simulink library "LIB_RTCP_DIE_UG_V1_0"  (R2021a)
settings: Solver=VariableStepAuto  StartTime=0.0  StopTime=10.0  RelTol=1e-3
undefined symbols (not defined in the file): DiscIntNeverNeededParam
libraries: c2802xlib x22, c28004xlib x10, pid_lib x2, spsAlphaBetaZerotodq0Lib x1, eeGeneralControl x1, eeStairGenerator x1
settings Model: Creator=luram  LastModifiedBy=luram

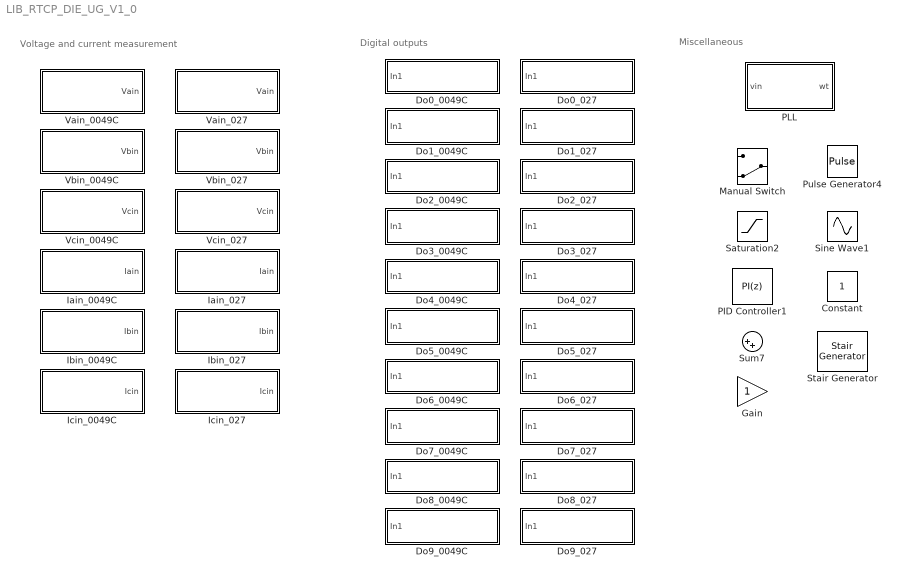
== system LIB_RTCP_DIE_UG_V1_0 ==
  note: Miscellaneous
  note: Digital outputs
  note: Voltage and current measurement
  Constant : Constant
  Do0_0049C : Subsystem
      mask Display: disp('\muC (boolean) --> Dout', 'texmode','on')
  Do0_027 : Subsystem
      mask Display: disp('\muC (boolean) --> Dout', 'texmode','on')
  Do1_0049C : Subsystem
      mask Display: disp('\muC (boolean) --> Dout', 'texmode','on')
  Do1_027 : Subsystem
      mask Display: disp('\muC (boolean) --> Dout', 'texmode','on')
  Do2_0049C : Subsystem
      mask Display: disp('\muC (boolean) --> Dout', 'texmode','on')
  Do2_027 : Subsystem
      mask Display: disp('\muC (boolean) --> Dout', 'texmode','on')
  Do3_0049C : Subsystem
      mask Display: disp('\muC (boolean) --> Dout', 'texmode','on')
  Do3_027 : Subsystem
      mask Display: disp('\muC (boolean) --> Dout', 'texmode','on')
  Do4_0049C : Subsystem
      mask Display: disp('\muC (boolean) --> Dout', 'texmode','on')
  Do4_027 : Subsystem
      mask Display: disp('\muC (boolean) --> Dout', 'texmode','on')
  Do5_0049C : Subsystem
      mask Display: disp('\muC (boolean) --> Dout', 'texmode','on')
  Do5_027 : Subsystem
      mask Display: disp('\muC (boolean) --> Dout', 'texmode','on')
  Do6_0049C : Subsystem
      mask Display: disp('\muC (boolean) --> Dout', 'texmode','on')
  Do6_027 : Subsystem
      mask Display: disp('\muC (boolean) --> Dout', 'texmode','on')
  Do7_0049C : Subsystem
      mask Display: disp('\muC (boolean) --> Dout', 'texmode','on')
  Do7_027 : Subsystem
      mask Display: disp('\muC (boolean) --> Dout', 'texmode','on')
  Do8_0049C : Subsystem
      mask Display: disp('\muC (boolean) --> Dout', 'texmode','on')
  Do8_027 : Subsystem
      mask Display: disp('\muC (boolean) --> Dout', 'texmode','on')
  Do9_0049C : Subsystem
      mask Display: disp('\muC (boolean) --> Dout', 'texmode','on')
  Do9_027 : Subsystem
      mask Display: disp('\muC (boolean) --> Dout', 'texmode','on')
  Gain : Gain
  Iain_0049C : Subsystem  mask(Voltage sensor){Off=0.15, AQPSv=50, Ts=1e-4}
      mask prompts: Off "Offset"; AQPSv "Adquisition"
      mask help:
      | R1=330;
      | R2=300e3;
      | Gain=8.2;
      | R2d=2000;
      | R1d=3000;
      |
      | GananciaAnV=R2d/R1d*Gain*R1/(R1+R2);
      | VtoD=GananciaAnV*4096/3.3;
      | DtoV=1/VtoD;
      mask init:
      | Gain=8.2;
      | R2d=2000;
      | R1d=3000;
      | 
      | Rs=0.02;
      | GananciaAnI=R2d/R1d*Gain*Rs;
      | ItoD=GananciaAnI*4096/3.3;
      | DtoI=1/ItoD;
      mask Help:
      | R1=330;
      | R2=300e3;
      | Gain=8.2;
      | R2d=2000;
      | R1d=3000;
      | 
      | GananciaAnV=R2d/R1d*Gain*R1/(R1+R2);
      | VtoD=GananciaAnV*4096/3.3;
      | DtoV=1/VtoD;
      mask Display: disp('Iin  --> \muC (single) ', 'texmode','on')
  Iain_027 : Subsystem  mask(Voltage sensor){Off=0.15, AQPSv=50, Ts=1e-4}
      mask prompts: Off "Offset"; AQPSv "Adquisition"
      mask help:
      | R1=330;
      | R2=300e3;
      | Gain=8.2;
      | R2d=2000;
      | R1d=3000;
      |
      | GananciaAnV=R2d/R1d*Gain*R1/(R1+R2);
      | VtoD=GananciaAnV*4096/3.3;
      | DtoV=1/VtoD;
      mask init:
      | Gain=8.2;
      | R2d=2000;
      | R1d=3000;
      | 
      | Rs=0.02;
      | GananciaAnI=R2d/R1d*Gain*Rs;
      | ItoD=GananciaAnI*4096/3.3;
      | DtoI=1/ItoD;
      mask Help:
      | R1=330;
      | R2=300e3;
      | Gain=8.2;
      | R2d=2000;
      | R1d=3000;
      | 
      | GananciaAnV=R2d/R1d*Gain*R1/(R1+R2);
      | VtoD=GananciaAnV*4096/3.3;
      | DtoV=1/VtoD;
      mask Display: disp('Iin  --> \muC (single) ', 'texmode','on')
  Ibin_0049C : Subsystem  mask(Voltage sensor){Off=0.15, AQPSv=50, Ts=1e-4}
      mask prompts: Off "Offset"; AQPSv "Adquisition"
      mask help:
      | R1=330;
      | R2=300e3;
      | Gain=8.2;
      | R2d=2000;
      | R1d=3000;
      |
      | GananciaAnV=R2d/R1d*Gain*R1/(R1+R2);
      | VtoD=GananciaAnV*4096/3.3;
      | DtoV=1/VtoD;
      mask init:
      | Gain=8.2;
      | R2d=2000;
      | R1d=3000;
      | 
      | Rs=0.02;
      | GananciaAnI=R2d/R1d*Gain*Rs;
      | ItoD=GananciaAnI*4096/3.3;
      | DtoI=1/ItoD;
      mask Help:
      | R1=330;
      | R2=300e3;
      | Gain=8.2;
      | R2d=2000;
      | R1d=3000;
      | 
      | GananciaAnV=R2d/R1d*Gain*R1/(R1+R2);
      | VtoD=GananciaAnV*4096/3.3;
      | DtoV=1/VtoD;
      mask Display: disp('Iin  --> \muC (single) ', 'texmode','on')
  Ibin_027 : Subsystem  mask(Voltage sensor){Off=0.15, AQPSv=50, Ts=1e-4}
      mask prompts: Off "Offset"; AQPSv "Adquisition"
      mask help:
      | R1=330;
      | R2=300e3;
      | Gain=8.2;
      | R2d=2000;
      | R1d=3000;
      |
      | GananciaAnV=R2d/R1d*Gain*R1/(R1+R2);
      | VtoD=GananciaAnV*4096/3.3;
      | DtoV=1/VtoD;
      mask init:
      | Gain=8.2;
      | R2d=2000;
      | R1d=3000;
      | 
      | Rs=0.02;
      | GananciaAnI=R2d/R1d*Gain*Rs;
      | ItoD=GananciaAnI*4096/3.3;
      | DtoI=1/ItoD;
      mask Help:
      | R1=330;
      | R2=300e3;
      | Gain=8.2;
      | R2d=2000;
      | R1d=3000;
      | 
      | GananciaAnV=R2d/R1d*Gain*R1/(R1+R2);
      | VtoD=GananciaAnV*4096/3.3;
      | DtoV=1/VtoD;
      mask Display: disp('Iin  --> \muC (single) ', 'texmode','on')
  Icin_0049C : Subsystem  mask(Voltage sensor){Off=0.15, AQPSv=50, Ts=1e-4}
      mask prompts: Off "Offset"; AQPSv "Adquisition"
      mask help:
      | R1=330;
      | R2=300e3;
      | Gain=8.2;
      | R2d=2000;
      | R1d=3000;
      |
      | GananciaAnV=R2d/R1d*Gain*R1/(R1+R2);
      | VtoD=GananciaAnV*4096/3.3;
      | DtoV=1/VtoD;
      mask init:
      | Gain=8.2;
      | R2d=2000;
      | R1d=3000;
      | 
      | Rs=0.02;
      | GananciaAnI=R2d/R1d*Gain*Rs;
      | ItoD=GananciaAnI*4096/3.3;
      | DtoI=1/ItoD;
      mask Help:
      | R1=330;
      | R2=300e3;
      | Gain=8.2;
      | R2d=2000;
      | R1d=3000;
      | 
      | GananciaAnV=R2d/R1d*Gain*R1/(R1+R2);
      | VtoD=GananciaAnV*4096/3.3;
      | DtoV=1/VtoD;
      mask Display: disp('Iin  --> \muC (single) ', 'texmode','on')
  Icin_027 : Subsystem  mask(Voltage sensor){Off=0.15, AQPSv=50, Ts=1e-4}
      mask prompts: Off "Offset"; AQPSv "Adquisition"
      mask help:
      | R1=330;
      | R2=300e3;
      | Gain=8.2;
      | R2d=2000;
      | R1d=3000;
      |
      | GananciaAnV=R2d/R1d*Gain*R1/(R1+R2);
      | VtoD=GananciaAnV*4096/3.3;
      | DtoV=1/VtoD;
      mask init:
      | Gain=8.2;
      | R2d=2000;
      | R1d=3000;
      | 
      | Rs=0.02;
      | GananciaAnI=R2d/R1d*Gain*Rs;
      | ItoD=GananciaAnI*4096/3.3;
      | DtoI=1/ItoD;
      mask Help:
      | R1=330;
      | R2=300e3;
      | Gain=8.2;
      | R2d=2000;
      | R1d=3000;
      | 
      | GananciaAnV=R2d/R1d*Gain*R1/(R1+R2);
      | VtoD=GananciaAnV*4096/3.3;
      | DtoV=1/VtoD;
      mask Display: disp('Iin  --> \muC (single) ', 'texmode','on')
  Manual Switch : ManualSwitch  CurrentSetting=0
  PID Controller1 : pid_lib/PID Controller  Controller=PI  Form=Parallel  TimeDomain=Discrete-time  UseExternalTs=off  SampleTime=1e-5  IntegratorMethod=Forward Euler  FilterMethod=Forward Euler  ControllerParametersSource=internal  P=1  I=1  D=0  UseFilter=on  N=100  TunerSelectOption=Transfer Function Based (PID Tuner App)  InitialConditionSource=internal  InitialConditionForIntegrator=0  InitialConditionForFilter=0  DifferentiatorICPrevScaledInput=0  ExternalReset=none  TrackingMode=off  Kt=1  LimitOutput=on  SatLimitsSource=internal  UpperSaturationLimit=1  LowerSaturationLimit=-1  LinearizeAsGain=on  AntiWindupMode=none  Kb=1  POutMin=[]  POutMax=[]  IOutMin=[]  IOutMax=[]  DOutMin=[]  DOutMax=[]  NOutMin=[]  NOutMax=[]  SumOutMin=[]  SumOutMax=[]  SaturationOutMin=[]  SaturationOutMax=[]  PParamMin=[]  PParamMax=[]  IParamMin=[]  IParamMax=[]  DParamMin=[]  DParamMax=[]  NParamMin=[]  NParamMax=[]  KbParamMin=[]  KbParamMax=[]  KtParamMin=[]  KtParamMax=[]  KbOutMin=[]  KbOutMax=[]  KtOutMin=[]  KtOutMax=[]  IntegratorOutMin=[]  IntegratorOutMax=[]  FilterOutMin=[]  FilterOutMax=[]  SumI1OutMin=[]  SumI1OutMax=[]  SumI2OutMin=[]  SumI2OutMax=[]  SumI3OutMin=[]  SumI3OutMax=[]  SumI4OutMin=[]  SumI4OutMax=[]  SumDOutMin=[]  SumDOutMax=[]  DifferentiatorOutMin=[]  DifferentiatorOutMax=[]  FilterDiffOutCoefMin=[]  FilterDiffOutCoefMax=[]  ReciprocalOutMin=[]  ReciprocalOutMax=[]  SumDenOutMin=[]  SumDenOutMax=[]  SumNumOutMin=[]  SumNumOutMax=[]  DivideOutMin=[]  DivideOutMax=[]  UdiffTsProdOutMin=[]  UdiffTsProdOutMax=[]  NTsProdOutMin=[]  NTsProdOutMax=[]  UintegralTsProdOutMin=[]  UintegralTsProdOutMax=[]  UngainTsProdOutMin=[]  UngainTsProdOutMax=[]  IntegratorContinuousStateAttributes=''  IntegratorStateMustResolveToSignalObject=off  IntegratorRTWStateStorageClass=Auto  FilterContinuousStateAttributes=''  FilterStateMustResolveToSignalObject=off  FilterRTWStateStorageClass=Auto  ParallelPVariant=InternalParameters  IdealPVariant=Disabled  IVariant=InternalParameters  DVariant=Disabled  IntegratorVariant=Discrete  SatVariant=Enabled  AWVariant=Passthrough  PCopyVariant=Disabled  TRVariant=Disabled  FdbkBlocksVariant=Forward  IdealPFdbkVariant=Disabled  SatFdbkVariant=Disabled  DerivativeFilterVariant=Disabled  NVariant=Disabled  NCopyVariant=Disabled_SignalSpec  FilterICVariant=Disabled  IntegratorICVariant=InternalICs  ExternalResetVariant=Disabled  TRSumVariant=Passthrough  SumFdbkVariant=Disabled  SumVariant=Sum_PI  TsampFilterVariant=InternalTs  TsampNgainVariant=Passthrough  TsampIntegralVariant=Passthrough  ExternalSaturationOutDataTypeStr=Inherit: Same as second input
  PLL : Subsystem  mask{Ffun=60, Ts=-1}
      mask prompts: Ffun "Fundamental Frequency"
      mask Display: disp('In  --> wt ', 'texmode','on')
  Pulse Generator4 : DiscretePulseGenerator  PulseType=Time based  Period=0.6  PulseWidth=50
  Saturation2 : Saturate  UpperLimit=4900  LowerLimit=100
  Sine Wave1 : Sin  Frequency=2*pi*60
  Stair Generator : eeStairGenerator/Stair Generator  LabelModeActiveChoice=Discrete  TimeInput=[0.5 1 3 3.5]  AmplitudeInput=[1 -1 2.5 0]  SampleTime=-1  RepeatPattern=off  OutDataTypeStr=double
      settings: SourceProductBaseCode=PS
  Sum7 : Sum  Inputs=|++
  Vain_0049C : Subsystem  mask(Voltage sensor){Off=3, AQPSv=50, Ts=1e-4}
      mask prompts: Off "Offset"; AQPSv "Adquisition"
      mask help:
      | R1=330;
      | R2=300e3;
      | Gain=8.2;
      | R2d=2000;
      | R1d=3000;
      |
      | GananciaAnV=R2d/R1d*Gain*R1/(R1+R2);
      | VtoD=GananciaAnV*4096/3.3;
      | DtoV=1/VtoD;
      mask init:
      | R1=330;
      | R2=300e3;
      | Gain=8.2;
      | R2d=2000;
      | R1d=3000;
      | 
      | GananciaAnV=R2d/R1d*Gain*R1/(R1+R2);
      | VtoD=GananciaAnV*4096/3.3;
      | DtoV=1/VtoD;
      mask Help:
      | R1=330;
      | R2=300e3;
      | Gain=8.2;
      | R2d=2000;
      | R1d=3000;
      | 
      | GananciaAnV=R2d/R1d*Gain*R1/(R1+R2);
      | VtoD=GananciaAnV*4096/3.3;
      | DtoV=1/VtoD;
      mask Display: disp('Vin  --> \muC (single) ', 'texmode','on')
  Vain_027 : Subsystem  mask(Voltage sensor){Off=3, AQPSv=50, Ts=1e-4}
      mask prompts: Off "Offset"; AQPSv "Adquisition"
      mask help:
      | R1=330;
      | R2=300e3;
      | Gain=8.2;
      | R2d=2000;
      | R1d=3000;
      |
      | GananciaAnV=R2d/R1d*Gain*R1/(R1+R2);
      | VtoD=GananciaAnV*4096/3.3;
      | DtoV=1/VtoD;
      mask init:
      | R1=330;
      | R2=300e3;
      | Gain=8.2;
      | R2d=2000;
      | R1d=3000;
      | 
      | GananciaAnV=R2d/R1d*Gain*R1/(R1+R2);
      | VtoD=GananciaAnV*4096/3.3;
      | DtoV=1/VtoD;
      mask Help:
      | R1=330;
      | R2=300e3;
      | Gain=8.2;
      | R2d=2000;
      | R1d=3000;
      | 
      | GananciaAnV=R2d/R1d*Gain*R1/(R1+R2);
      | VtoD=GananciaAnV*4096/3.3;
      | DtoV=1/VtoD;
      mask Display: disp('Vin  --> \muC (single) ', 'texmode','on')
  Vbin_0049C : Subsystem  mask{Off=3, AQPSv=50, Ts=1e-4}
      mask prompts: Off "Offset"; AQPSv "Adquisition"
      mask init:
      | R1=330;
      | R2=300e3;
      | Gain=8.2;
      | R2d=2000;
      | R1d=3000;
      | 
      | GananciaAnV=R2d/R1d*Gain*R1/(R1+R2);
      | VtoD=GananciaAnV*4096/3.3;
      | DtoV=1/VtoD;
      mask Display: disp('Vin  --> \muC (single) ', 'texmode','on')
  Vbin_027 : Subsystem  mask{Off=3, AQPSv=50, Ts=1e-4}
      mask prompts: Off "Offset"; AQPSv "Adquisition"
      mask init:
      | R1=330;
      | R2=300e3;
      | Gain=8.2;
      | R2d=2000;
      | R1d=3000;
      | 
      | GananciaAnV=R2d/R1d*Gain*R1/(R1+R2);
      | VtoD=GananciaAnV*4096/3.3;
      | DtoV=1/VtoD;
      mask Display: disp('Vin  --> \muC (single) ', 'texmode','on')
  Vcin_0049C : Subsystem  mask{Off=3, AQPSv=50, Ts=1e-4}
      mask prompts: Off "Offset"; AQPSv "Adquisition"
      mask init:
      | R1=330;
      | R2=300e3;
      | Gain=8.2;
      | R2d=2000;
      | R1d=3000;
      | 
      | GananciaAnV=R2d/R1d*Gain*R1/(R1+R2);
      | VtoD=GananciaAnV*4096/3.3;
      | DtoV=1/VtoD;
      mask Display: disp('Vin  --> \muC (single) ', 'texmode','on')
  Vcin_027 : Subsystem  mask{Off=3, AQPSv=50, Ts=1e-4}
      mask prompts: Off "Offset"; AQPSv "Adquisition"
      mask init:
      | R1=330;
      | R2=300e3;
      | Gain=8.2;
      | R2d=2000;
      | R1d=3000;
      | 
      | GananciaAnV=R2d/R1d*Gain*R1/(R1+R2);
      | VtoD=GananciaAnV*4096/3.3;
      | DtoV=1/VtoD;
      mask Display: disp('Vin  --> \muC (single) ', 'texmode','on')

== system LIB_RTCP_DIE_UG_V1_0/Do0_0049C ==
  In1 : Inport
  Digital Output : c28004xlib/Digital Output  GPIO_Number=GPIO8~GPIO15  GPIO_Bit0=off  GPIO_BIT0_Toggle=off  GPIO_Bit1=off  GPIO_BIT1_Toggle=off  GPIO_Bit2=on  GPIO_BIT2_Toggle=off  GPIO_Bit3=off  GPIO_BIT3_Toggle=off  GPIO_Bit4=off  GPIO_BIT4_Toggle=off  GPIO_Bit5=off  GPIO_BIT5_Toggle=off  GPIO_Bit6=off  GPIO_BIT6_Toggle=off  GPIO_Bit7=off  GPIO_BIT7_Toggle=off
      settings: SourceProductBaseCode=TIC2000
  wires:
  In1/1 -> Digital Output/1

== system LIB_RTCP_DIE_UG_V1_0/Do0_027 ==
  In1 : Inport
  Digital Output : c2802xlib/Digital Output  GPIO_Number=GPIO0~GPIO7  GPIO_Bit0=on  GPIO_BIT0_Toggle=off  GPIO_Bit1=off  GPIO_BIT1_Toggle=off  GPIO_Bit2=off  GPIO_BIT2_Toggle=off  GPIO_Bit3=off  GPIO_BIT3_Toggle=off  GPIO_Bit4=off  GPIO_BIT4_Toggle=off  GPIO_Bit5=off  GPIO_BIT5_Toggle=off  GPIO_Bit6=off  GPIO_BIT6_Toggle=off  GPIO_Bit7=off  GPIO_BIT7_Toggle=off
      settings: SourceProductBaseCode=TIC2000
  wires:
  In1/1 -> Digital Output/1

== system LIB_RTCP_DIE_UG_V1_0/Do1_0049C ==
  In1 : Inport
  Digital Output : c28004xlib/Digital Output  GPIO_Number=GPIO8~GPIO15  GPIO_Bit0=off  GPIO_BIT0_Toggle=off  GPIO_Bit1=off  GPIO_BIT1_Toggle=off  GPIO_Bit2=off  GPIO_BIT2_Toggle=off  GPIO_Bit3=on  GPIO_BIT3_Toggle=off  GPIO_Bit4=off  GPIO_BIT4_Toggle=off  GPIO_Bit5=off  GPIO_BIT5_Toggle=off  GPIO_Bit6=off  GPIO_BIT6_Toggle=off  GPIO_Bit7=off  GPIO_BIT7_Toggle=off
      settings: SourceProductBaseCode=TIC2000
  wires:
  In1/1 -> Digital Output/1

== system LIB_RTCP_DIE_UG_V1_0/Do1_027 ==
  In1 : Inport
  Digital Output : c2802xlib/Digital Output  GPIO_Number=GPIO0~GPIO7  GPIO_Bit0=off  GPIO_BIT0_Toggle=off  GPIO_Bit1=on  GPIO_BIT1_Toggle=off  GPIO_Bit2=off  GPIO_BIT2_Toggle=off  GPIO_Bit3=off  GPIO_BIT3_Toggle=off  GPIO_Bit4=off  GPIO_BIT4_Toggle=off  GPIO_Bit5=off  GPIO_BIT5_Toggle=off  GPIO_Bit6=off  GPIO_BIT6_Toggle=off  GPIO_Bit7=off  GPIO_BIT7_Toggle=off
      settings: SourceProductBaseCode=TIC2000
  wires:
  In1/1 -> Digital Output/1

== system LIB_RTCP_DIE_UG_V1_0/Do2_0049C ==
  In1 : Inport
  Digital Output : c28004xlib/Digital Output  GPIO_Number=GPIO8~GPIO15  GPIO_Bit0=on  GPIO_BIT0_Toggle=off  GPIO_Bit1=off  GPIO_BIT1_Toggle=off  GPIO_Bit2=off  GPIO_BIT2_Toggle=off  GPIO_Bit3=off  GPIO_BIT3_Toggle=off  GPIO_Bit4=off  GPIO_BIT4_Toggle=off  GPIO_Bit5=off  GPIO_BIT5_Toggle=off  GPIO_Bit6=off  GPIO_BIT6_Toggle=off  GPIO_Bit7=off  GPIO_BIT7_Toggle=off
      settings: SourceProductBaseCode=TIC2000
  wires:
  In1/1 -> Digital Output/1

== system LIB_RTCP_DIE_UG_V1_0/Do2_027 ==
  In1 : Inport
  Digital Output : c2802xlib/Digital Output  GPIO_Number=GPIO0~GPIO7  GPIO_Bit0=off  GPIO_BIT0_Toggle=off  GPIO_Bit1=off  GPIO_BIT1_Toggle=off  GPIO_Bit2=on  GPIO_BIT2_Toggle=off  GPIO_Bit3=off  GPIO_BIT3_Toggle=off  GPIO_Bit4=off  GPIO_BIT4_Toggle=off  GPIO_Bit5=off  GPIO_BIT5_Toggle=off  GPIO_Bit6=off  GPIO_BIT6_Toggle=off  GPIO_Bit7=off  GPIO_BIT7_Toggle=off
      settings: SourceProductBaseCode=TIC2000
  wires:
  In1/1 -> Digital Output/1

== system LIB_RTCP_DIE_UG_V1_0/Do3_0049C ==
  In1 : Inport
  Digital Output : c28004xlib/Digital Output  GPIO_Number=GPIO8~GPIO15  GPIO_Bit0=off  GPIO_BIT0_Toggle=off  GPIO_Bit1=on  GPIO_BIT1_Toggle=off  GPIO_Bit2=off  GPIO_BIT2_Toggle=off  GPIO_Bit3=off  GPIO_BIT3_Toggle=off  GPIO_Bit4=off  GPIO_BIT4_Toggle=off  GPIO_Bit5=off  GPIO_BIT5_Toggle=off  GPIO_Bit6=off  GPIO_BIT6_Toggle=off  GPIO_Bit7=off  GPIO_BIT7_Toggle=off
      settings: SourceProductBaseCode=TIC2000
  wires:
  In1/1 -> Digital Output/1

== system LIB_RTCP_DIE_UG_V1_0/Do3_027 ==
  In1 : Inport
  Digital Output : c2802xlib/Digital Output  GPIO_Number=GPIO0~GPIO7  GPIO_Bit0=off  GPIO_BIT0_Toggle=off  GPIO_Bit1=off  GPIO_BIT1_Toggle=off  GPIO_Bit2=off  GPIO_BIT2_Toggle=off  GPIO_Bit3=on  GPIO_BIT3_Toggle=off  GPIO_Bit4=off  GPIO_BIT4_Toggle=off  GPIO_Bit5=off  GPIO_BIT5_Toggle=off  GPIO_Bit6=off  GPIO_BIT6_Toggle=off  GPIO_Bit7=off  GPIO_BIT7_Toggle=off
      settings: SourceProductBaseCode=TIC2000
  wires:
  In1/1 -> Digital Output/1

== system LIB_RTCP_DIE_UG_V1_0/Do4_0049C ==
  In1 : Inport
  Digital Output : c28004xlib/Digital Output  GPIO_Number=GPIO0~GPIO7  GPIO_Bit0=off  GPIO_BIT0_Toggle=off  GPIO_Bit1=off  GPIO_BIT1_Toggle=off  GPIO_Bit2=off  GPIO_BIT2_Toggle=off  GPIO_Bit3=off  GPIO_BIT3_Toggle=off  GPIO_Bit4=on  GPIO_BIT4_Toggle=off  GPIO_Bit5=off  GPIO_BIT5_Toggle=off  GPIO_Bit6=off  GPIO_BIT6_Toggle=off  GPIO_Bit7=off  GPIO_BIT7_Toggle=off
      settings: SourceProductBaseCode=TIC2000
  wires:
  In1/1 -> Digital Output/1

== system LIB_RTCP_DIE_UG_V1_0/Do4_027 ==
  In1 : Inport
  Digital Output : c2802xlib/Digital Output  GPIO_Number=GPIO0~GPIO7  GPIO_Bit0=off  GPIO_BIT0_Toggle=off  GPIO_Bit1=off  GPIO_BIT1_Toggle=off  GPIO_Bit2=off  GPIO_BIT2_Toggle=off  GPIO_Bit3=off  GPIO_BIT3_Toggle=off  GPIO_Bit4=on  GPIO_BIT4_Toggle=off  GPIO_Bit5=off  GPIO_BIT5_Toggle=off  GPIO_Bit6=off  GPIO_BIT6_Toggle=off  GPIO_Bit7=off  GPIO_BIT7_Toggle=off
      settings: SourceProductBaseCode=TIC2000
  wires:
  In1/1 -> Digital Output/1

== system LIB_RTCP_DIE_UG_V1_0/Do5_0049C ==
  In1 : Inport
  Digital Output : c28004xlib/Digital Output  GPIO_Number=GPIO0~GPIO7  GPIO_Bit0=off  GPIO_BIT0_Toggle=off  GPIO_Bit1=off  GPIO_BIT1_Toggle=off  GPIO_Bit2=off  GPIO_BIT2_Toggle=off  GPIO_Bit3=off  GPIO_BIT3_Toggle=off  GPIO_Bit4=off  GPIO_BIT4_Toggle=off  GPIO_Bit5=on  GPIO_BIT5_Toggle=off  GPIO_Bit6=off  GPIO_BIT6_Toggle=off  GPIO_Bit7=off  GPIO_BIT7_Toggle=off
      settings: SourceProductBaseCode=TIC2000
  wires:
  In1/1 -> Digital Output/1

== system LIB_RTCP_DIE_UG_V1_0/Do5_027 ==
  In1 : Inport
  Digital Output : c2802xlib/Digital Output  GPIO_Number=GPIO0~GPIO7  GPIO_Bit0=off  GPIO_BIT0_Toggle=off  GPIO_Bit1=off  GPIO_BIT1_Toggle=off  GPIO_Bit2=off  GPIO_BIT2_Toggle=off  GPIO_Bit3=off  GPIO_BIT3_Toggle=off  GPIO_Bit4=off  GPIO_BIT4_Toggle=off  GPIO_Bit5=on  GPIO_BIT5_Toggle=off  GPIO_Bit6=off  GPIO_BIT6_Toggle=off  GPIO_Bit7=off  GPIO_BIT7_Toggle=off
      settings: SourceProductBaseCode=TIC2000
  wires:
  In1/1 -> Digital Output/1

== system LIB_RTCP_DIE_UG_V1_0/Do6_0049C ==
  In1 : Inport
  Digital Output : c28004xlib/Digital Output  GPIO_Number=GPIO16~GPIO23  GPIO_Bit0=on  GPIO_BIT0_Toggle=off  GPIO_Bit1=off  GPIO_BIT1_Toggle=off  GPIO_Bit2=off  GPIO_BIT2_Toggle=off  GPIO_Bit3=off  GPIO_BIT3_Toggle=off  GPIO_Bit4=off  GPIO_BIT4_Toggle=off  GPIO_Bit5=off  GPIO_BIT5_Toggle=off  GPIO_Bit6=off  GPIO_BIT6_Toggle=off  GPIO_Bit7=off  GPIO_BIT7_Toggle=off
      settings: SourceProductBaseCode=TIC2000
  wires:
  In1/1 -> Digital Output/1

== system LIB_RTCP_DIE_UG_V1_0/Do6_027 ==
  In1 : Inport
  Digital Output : c2802xlib/Digital Output  GPIO_Number=GPIO0~GPIO7  GPIO_Bit0=off  GPIO_BIT0_Toggle=off  GPIO_Bit1=off  GPIO_BIT1_Toggle=off  GPIO_Bit2=off  GPIO_BIT2_Toggle=off  GPIO_Bit3=off  GPIO_BIT3_Toggle=off  GPIO_Bit4=off  GPIO_BIT4_Toggle=off  GPIO_Bit5=off  GPIO_BIT5_Toggle=off  GPIO_Bit6=on  GPIO_BIT6_Toggle=off  GPIO_Bit7=off  GPIO_BIT7_Toggle=off
      settings: SourceProductBaseCode=TIC2000
  wires:
  In1/1 -> Digital Output/1

== system LIB_RTCP_DIE_UG_V1_0/Do7_0049C ==
  In1 : Inport
  Digital Output : c28004xlib/Digital Output  GPIO_Number=GPIO16~GPIO23  GPIO_Bit0=off  GPIO_BIT0_Toggle=off  GPIO_Bit1=on  GPIO_BIT1_Toggle=off  GPIO_Bit2=off  GPIO_BIT2_Toggle=off  GPIO_Bit3=off  GPIO_BIT3_Toggle=off  GPIO_Bit4=off  GPIO_BIT4_Toggle=off  GPIO_Bit5=off  GPIO_BIT5_Toggle=off  GPIO_Bit6=off  GPIO_BIT6_Toggle=off  GPIO_Bit7=off  GPIO_BIT7_Toggle=off
      settings: SourceProductBaseCode=TIC2000
  wires:
  In1/1 -> Digital Output/1

== system LIB_RTCP_DIE_UG_V1_0/Do7_027 ==
  In1 : Inport
  Digital Output : c2802xlib/Digital Output  GPIO_Number=GPIO0~GPIO7  GPIO_Bit0=off  GPIO_BIT0_Toggle=off  GPIO_Bit1=off  GPIO_BIT1_Toggle=off  GPIO_Bit2=off  GPIO_BIT2_Toggle=off  GPIO_Bit3=off  GPIO_BIT3_Toggle=off  GPIO_Bit4=off  GPIO_BIT4_Toggle=off  GPIO_Bit5=off  GPIO_BIT5_Toggle=off  GPIO_Bit6=off  GPIO_BIT6_Toggle=off  GPIO_Bit7=on  GPIO_BIT7_Toggle=off
      settings: SourceProductBaseCode=TIC2000
  wires:
  In1/1 -> Digital Output/1

== system LIB_RTCP_DIE_UG_V1_0/Do8_0049C ==
  In1 : Inport
  Digital Output : c28004xlib/Digital Output  GPIO_Number=GPIO56~GPIO63  GPIO_Bit0=off  GPIO_BIT0_Toggle=off  GPIO_Bit1=off  GPIO_BIT1_Toggle=off  GPIO_Bit2=on  GPIO_BIT2_Toggle=off  GPIO_Bit3=off  GPIO_BIT3_Toggle=off  GPIO_Bit4=off  GPIO_BIT4_Toggle=off  GPIO_Bit5=off  GPIO_BIT5_Toggle=off  GPIO_Bit6=off  GPIO_BIT6_Toggle=off  GPIO_Bit7=off  GPIO_BIT7_Toggle=off
      settings: SourceProductBaseCode=TIC2000
  wires:
  In1/1 -> Digital Output/1

== system LIB_RTCP_DIE_UG_V1_0/Do8_027 ==
  In1 : Inport
  Digital Output : c2802xlib/Digital Output  GPIO_Number=GPIO16~GPIO23  GPIO_Bit0=on  GPIO_BIT0_Toggle=off  GPIO_Bit1=off  GPIO_BIT1_Toggle=off  GPIO_Bit2=off  GPIO_BIT2_Toggle=off  GPIO_Bit3=off  GPIO_BIT3_Toggle=off  GPIO_Bit4=off  GPIO_BIT4_Toggle=off  GPIO_Bit5=off  GPIO_BIT5_Toggle=off  GPIO_Bit6=off  GPIO_BIT6_Toggle=off  GPIO_Bit7=off  GPIO_BIT7_Toggle=off
      settings: SourceProductBaseCode=TIC2000
  wires:
  In1/1 -> Digital Output/1

== system LIB_RTCP_DIE_UG_V1_0/Do9_0049C ==
  In1 : Inport
  Digital Output : c28004xlib/Digital Output  GPIO_Number=GPIO24~GPIO31  GPIO_Bit0=off  GPIO_BIT0_Toggle=off  GPIO_Bit1=off  GPIO_BIT1_Toggle=off  GPIO_Bit2=off  GPIO_BIT2_Toggle=off  GPIO_Bit3=off  GPIO_BIT3_Toggle=off  GPIO_Bit4=off  GPIO_BIT4_Toggle=off  GPIO_Bit5=off  GPIO_BIT5_Toggle=off  GPIO_Bit6=on  GPIO_BIT6_Toggle=off  GPIO_Bit7=off  GPIO_BIT7_Toggle=off
      settings: SourceProductBaseCode=TIC2000
  wires:
  In1/1 -> Digital Output/1

== system LIB_RTCP_DIE_UG_V1_0/Do9_027 ==
  In1 : Inport
  Digital Output : c2802xlib/Digital Output  GPIO_Number=GPIO16~GPIO23  GPIO_Bit0=off  GPIO_BIT0_Toggle=off  GPIO_Bit1=on  GPIO_BIT1_Toggle=off  GPIO_Bit2=off  GPIO_BIT2_Toggle=off  GPIO_Bit3=off  GPIO_BIT3_Toggle=off  GPIO_Bit4=off  GPIO_BIT4_Toggle=off  GPIO_Bit5=off  GPIO_BIT5_Toggle=off  GPIO_Bit6=off  GPIO_BIT6_Toggle=off  GPIO_Bit7=off  GPIO_BIT7_Toggle=off
      settings: SourceProductBaseCode=TIC2000
  wires:
  In1/1 -> Digital Output/1

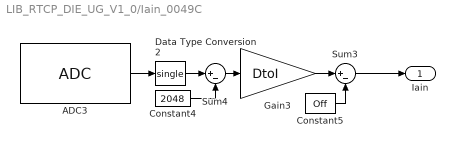
== system LIB_RTCP_DIE_UG_V1_0/Iain_0049C ==
  ADC3 : c2802xlib/ADC  blkParamProc=C2000_Type5  ADCModule=B  samplingMode=Single sample mode  ADCResolution=12-bit (Single-ended input)  useSOC1=SOC1  useSOC2=SOC0_SOC1  SOCAcquisitionWindow=AQPSv  SOCTriggerSource=Software  SOCInterruptTrigger=No ADCINT  Ts=Ts  dType=uint16  postInterrupt=off  interruptSel=ADCINT1  ADCINTContinuous=on  endma=off  chdma=1  conv1=ADCINA0  conv2=ADCINA0 and ADCINB0  conv1_Type4=ADCIN2  conv2_Type4=ADCIN0 and ADCIN1
  Constant4 : Constant  Value=2048
  Constant5 : Constant  Value=Off
  Data Type Conversion2 : DataTypeConversion  OutDataTypeStr=single
  Gain3 : Gain  Gain=DtoI
  Sum3 : Sum  Inputs=|+-
  Sum4 : Sum  Inputs=|+-
  Iain : Outport
  wires:
  Sum4/1 -> Gain3/1
  Sum3/1 -> Iain/1
  Gain3/1 -> Sum3/1
  Constant4/1 -> Sum4/2
  Constant5/1 -> Sum3/2
  Data Type Conversion2/1 -> Sum4/1
  ADC3/1 -> Data Type Conversion2/1

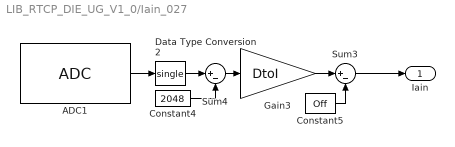
== system LIB_RTCP_DIE_UG_V1_0/Iain_027 ==
  ADC1 : c2802xlib/ADC  blkParamProc=C2000  ADCModule=1  samplingMode=Single sample mode  ADCResolution=12-bit (Single-ended input)  useSOC1=SOC0  useSOC2=SOC0_SOC1  SOCAcquisitionWindow=AQPSv  SOCTriggerSource=Software  SOCInterruptTrigger=No ADCINT  Ts=Ts  dType=uint16  postInterrupt=off  interruptSel=ADCINT1  ADCINTContinuous=on  endma=off  chdma=1  conv1=ADCINB1  conv2=ADCINA0 and ADCINB0  conv1_Type4=ADCIN0  conv2_Type4=ADCIN0 and ADCIN1
  Constant4 : Constant  Value=2048
  Constant5 : Constant  Value=Off
  Data Type Conversion2 : DataTypeConversion  OutDataTypeStr=single
  Gain3 : Gain  Gain=DtoI
  Sum3 : Sum  Inputs=|+-
  Sum4 : Sum  Inputs=|+-
  Iain : Outport
  wires:
  Sum4/1 -> Gain3/1
  Sum3/1 -> Iain/1
  Gain3/1 -> Sum3/1
  Constant4/1 -> Sum4/2
  Constant5/1 -> Sum3/2
  Data Type Conversion2/1 -> Sum4/1
  ADC1/1 -> Data Type Conversion2/1

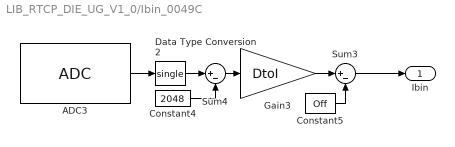
== system LIB_RTCP_DIE_UG_V1_0/Ibin_0049C ==
  ADC3 : c2802xlib/ADC  blkParamProc=C2000_Type5  ADCModule=C  samplingMode=Single sample mode  ADCResolution=12-bit (Single-ended input)  useSOC1=SOC1  useSOC2=SOC0_SOC1  SOCAcquisitionWindow=AQPSv  SOCTriggerSource=Software  SOCInterruptTrigger=No ADCINT  Ts=Ts  dType=uint16  postInterrupt=off  interruptSel=ADCINT1  ADCINTContinuous=on  endma=off  chdma=1  conv1=ADCINA0  conv2=ADCINA0 and ADCINB0  conv1_Type4=ADCIN0  conv2_Type4=ADCIN0 and ADCIN1
  Constant4 : Constant  Value=2048
  Constant5 : Constant  Value=Off
  Data Type Conversion2 : DataTypeConversion  OutDataTypeStr=single
  Gain3 : Gain  Gain=DtoI
  Sum3 : Sum  Inputs=|+-
  Sum4 : Sum  Inputs=|+-
  Ibin : Outport
  wires:
  Sum4/1 -> Gain3/1
  Sum3/1 -> Ibin/1
  Gain3/1 -> Sum3/1
  Constant4/1 -> Sum4/2
  Constant5/1 -> Sum3/2
  Data Type Conversion2/1 -> Sum4/1
  ADC3/1 -> Data Type Conversion2/1

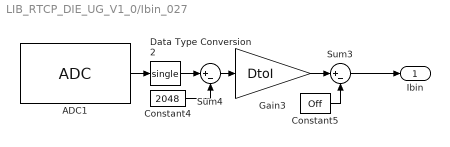
== system LIB_RTCP_DIE_UG_V1_0/Ibin_027 ==
  ADC1 : c2802xlib/ADC  blkParamProc=C2000  ADCModule=1  samplingMode=Single sample mode  ADCResolution=12-bit (Single-ended input)  useSOC1=SOC0  useSOC2=SOC0_SOC1  SOCAcquisitionWindow=AQPSv  SOCTriggerSource=Software  SOCInterruptTrigger=No ADCINT  Ts=Ts  dType=uint16  postInterrupt=off  interruptSel=ADCINT1  ADCINTContinuous=on  endma=off  chdma=1  conv1=ADCINB3  conv2=ADCINA0 and ADCINB0  conv1_Type4=ADCIN0  conv2_Type4=ADCIN0 and ADCIN1
  Constant4 : Constant  Value=2048
  Constant5 : Constant  Value=Off
  Data Type Conversion2 : DataTypeConversion  OutDataTypeStr=single
  Gain3 : Gain  Gain=DtoI
  Sum3 : Sum  Inputs=|+-
  Sum4 : Sum  Inputs=|+-
  Ibin : Outport
  wires:
  Sum4/1 -> Gain3/1
  Sum3/1 -> Ibin/1
  Gain3/1 -> Sum3/1
  Constant4/1 -> Sum4/2
  Constant5/1 -> Sum3/2
  Data Type Conversion2/1 -> Sum4/1
  ADC1/1 -> Data Type Conversion2/1

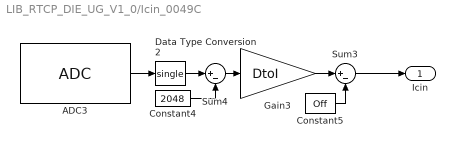
== system LIB_RTCP_DIE_UG_V1_0/Icin_0049C ==
  ADC3 : c2802xlib/ADC  blkParamProc=C2000_Type5  ADCModule=A  samplingMode=Single sample mode  ADCResolution=12-bit (Single-ended input)  useSOC1=SOC1  useSOC2=SOC0_SOC1  SOCAcquisitionWindow=AQPSv  SOCTriggerSource=Software  SOCInterruptTrigger=No ADCINT  Ts=Ts  dType=uint16  postInterrupt=off  interruptSel=ADCINT1  ADCINTContinuous=on  endma=off  chdma=1  conv1=ADCINA0  conv2=ADCINA0 and ADCINB0  conv1_Type4=ADCIN9  conv2_Type4=ADCIN0 and ADCIN1
  Constant4 : Constant  Value=2048
  Constant5 : Constant  Value=Off
  Data Type Conversion2 : DataTypeConversion  OutDataTypeStr=single
  Gain3 : Gain  Gain=DtoI
  Sum3 : Sum  Inputs=|+-
  Sum4 : Sum  Inputs=|+-
  Icin : Outport
  wires:
  Sum4/1 -> Gain3/1
  Sum3/1 -> Icin/1
  Gain3/1 -> Sum3/1
  Constant4/1 -> Sum4/2
  Constant5/1 -> Sum3/2
  Data Type Conversion2/1 -> Sum4/1
  ADC3/1 -> Data Type Conversion2/1

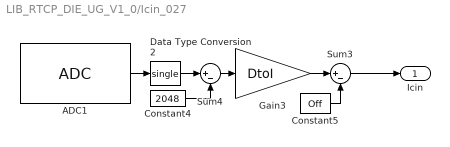
== system LIB_RTCP_DIE_UG_V1_0/Icin_027 ==
  ADC1 : c2802xlib/ADC  blkParamProc=C2000  ADCModule=1  samplingMode=Single sample mode  ADCResolution=12-bit (Single-ended input)  useSOC1=SOC0  useSOC2=SOC0_SOC1  SOCAcquisitionWindow=AQPSv  SOCTriggerSource=Software  SOCInterruptTrigger=No ADCINT  Ts=Ts  dType=uint16  postInterrupt=off  interruptSel=ADCINT1  ADCINTContinuous=on  endma=off  chdma=1  conv1=ADCINB7  conv2=ADCINA0 and ADCINB0  conv1_Type4=ADCIN0  conv2_Type4=ADCIN0 and ADCIN1
  Constant4 : Constant  Value=2048
  Constant5 : Constant  Value=Off
  Data Type Conversion2 : DataTypeConversion  OutDataTypeStr=single
  Gain3 : Gain  Gain=DtoI
  Sum3 : Sum  Inputs=|+-
  Sum4 : Sum  Inputs=|+-
  Icin : Outport
  wires:
  Sum4/1 -> Gain3/1
  Sum3/1 -> Icin/1
  Gain3/1 -> Sum3/1
  Constant4/1 -> Sum4/2
  Constant5/1 -> Sum3/2
  Data Type Conversion2/1 -> Sum4/1
  ADC1/1 -> Data Type Conversion2/1

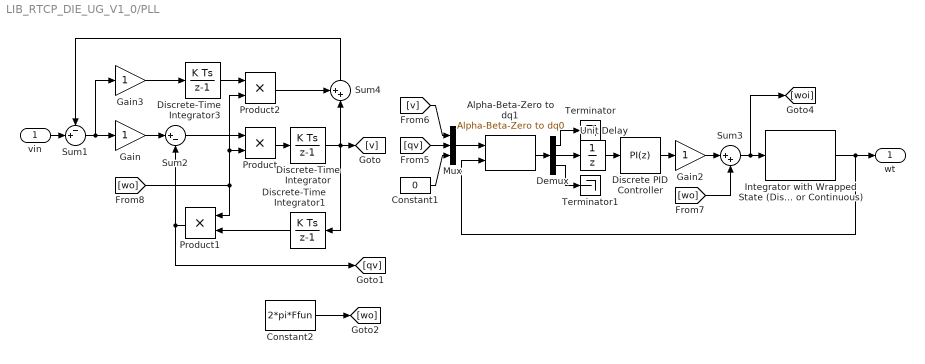
== system LIB_RTCP_DIE_UG_V1_0/PLL ==
  vin : Inport
  Alpha-Beta-Zero to dq1 : spsAlphaBetaZerotodq0Lib/Alpha-Beta-Zero to dq0  Alignment=90 degrees behind phase A axis
      settings: SourceProductBaseCode=PS
  Constant1 : Constant  Value=0
  Constant2 : Constant  Value=2*pi*Ffun
  Demux : Demux  Outputs=3
  Discrete PID Controller : pid_lib/PID Controller  Controller=PI  Form=Parallel  TimeDomain=Discrete-time  UseExternalTs=off  SampleTime=Ts  IntegratorMethod=Forward Euler  FilterMethod=Forward Euler  ControllerParametersSource=internal  P=1  I=1  D=0  UseFilter=on  N=100  TunerSelectOption=Transfer Function Based (PID Tuner App)  ZeroCross=off  InitialConditionSource=internal  InitialConditionForIntegrator=0  InitialConditionForFilter=0  DifferentiatorICPrevScaledInput=0  ExternalReset=none  TrackingMode=off  Kt=1  LimitOutput=on  SatLimitsSource=internal  UpperSaturationLimit=inf  LowerSaturationLimit=-inf  LinearizeAsGain=off  AntiWindupMode=back-calculation  Kb=1  POutMin=[]  POutMax=[]  IOutMin=[]  IOutMax=[]  DOutMin=[]  DOutMax=[]  NOutMin=[]  NOutMax=[]  SumOutMin=[]  SumOutMax=[]  SaturationOutMin=[]  SaturationOutMax=[]  PParamMin=[]  PParamMax=[]  IParamMin=[]  IParamMax=[]  DParamMin=[]  DParamMax=[]  NParamMin=[]  NParamMax=[]  KbParamMin=[]  KbParamMax=[]  KtParamMin=[]  KtParamMax=[]  KbOutMin=[]  KbOutMax=[]  KtOutMin=[]  KtOutMax=[]  IntegratorOutMin=[]  IntegratorOutMax=[]  FilterOutMin=[]  FilterOutMax=[]  SumI1OutMin=[]  SumI1OutMax=[]  SumI2OutMin=[]  SumI2OutMax=[]  SumI3OutMin=[]  SumI3OutMax=[]  SumI4OutMin=[]  SumI4OutMax=[]  SumDOutMin=[]  SumDOutMax=[]  DifferentiatorOutMin=[]  DifferentiatorOutMax=[]  FilterDiffOutCoefMin=[]  FilterDiffOutCoefMax=[]  ReciprocalOutMin=[]  ReciprocalOutMax=[]  SumDenOutMin=[]  SumDenOutMax=[]  SumNumOutMin=[]  SumNumOutMax=[]  DivideOutMin=[]  DivideOutMax=[]  UdiffTsProdOutMin=[]  UdiffTsProdOutMax=[]  NTsProdOutMin=[]  NTsProdOutMax=[]  UintegralTsProdOutMin=[]  UintegralTsProdOutMax=[]  UngainTsProdOutMin=[]  UngainTsProdOutMax=[]  IntegratorContinuousStateAttributes=''  IntegratorStateMustResolveToSignalObject=off  IntegratorRTWStateStorageClass=Auto  FilterContinuousStateAttributes=''  FilterStateMustResolveToSignalObject=off  FilterRTWStateStorageClass=Auto  ParallelPVariant=InternalParameters  IdealPVariant=Disabled  IVariant=InternalParameters  DVariant=Disabled  IntegratorVariant=Discrete  SatVariant=Enabled  AWVariant=BackCalculation  PCopyVariant=Disabled  TRVariant=Disabled  FdbkBlocksVariant=Forward  IdealPFdbkVariant=Disabled  SatFdbkVariant=Disabled  DerivativeFilterVariant=Disabled  NVariant=Disabled  NCopyVariant=Disabled_SignalSpec  FilterICVariant=Disabled  IntegratorICVariant=InternalICs  ExternalResetVariant=Disabled  TRSumVariant=Passthrough  SumFdbkVariant=Disabled  SumVariant=Sum_PI  TsampFilterVariant=InternalTs  TsampNgainVariant=Passthrough  TsampIntegralVariant=Passthrough  ExternalSaturationOutDataTypeStr=Inherit: Same as second input
  Discrete-Time Integrator : DiscreteIntegrator  SampleTime=Ts  ICPrevOutput=DiscIntNeverNeededParam  ICPrevScaledInput=DiscIntNeverNeededParam
  Discrete-Time Integrator1 : DiscreteIntegrator  SampleTime=Ts  ICPrevOutput=DiscIntNeverNeededParam  ICPrevScaledInput=DiscIntNeverNeededParam
  Discrete-Time Integrator3 : DiscreteIntegrator  SampleTime=Ts  ICPrevOutput=DiscIntNeverNeededParam  ICPrevScaledInput=DiscIntNeverNeededParam
  Gain : Gain
  Gain2 : Gain
  Gain3 : Gain
  Integrator with Wrapped State (Discrete or Continuous) : eeGeneralControl/Integrator with Wrapped State (Discrete or Continuous)  LabelModeActiveChoice=Discrete  WrappedStateUpperValue=2*pi  WrappedStateLowerValue=0  x0=0  Ts=Ts
      settings: SourceProductBaseCode=PS
  Mux : Mux  Inputs=3
  Product : Product
  Product1 : Product
  Product2 : Product
  Sum1 : Sum  Inputs=-+|
  Sum2 : Sum  Inputs=|+-
  Sum3 : Sum  Inputs=|++
  Sum4 : Sum  Inputs=++|
  Terminator : Terminator
  Terminator1 : Terminator
  Unit Delay : UnitDelay  SampleTime=-1  HasFrameUpgradeWarning=on
  wt : Outport
  wires:
  Discrete-Time Integrator/1 -> Sum4/2, [v], Discrete-Time Integrator1/1
  [wo] -> Product2/2, Product/2, Product1/1
  Product1/1 -> [qv], Sum2/2
  Discrete-Time Integrator1/1 -> Product1/2
  Integrator with Wrapped State (Discrete or Continuous)/1 -> Alpha-Beta-Zero to dq1/2, wt/1
  Demux/1 -> Terminator/1
  Gain/1 -> Sum2/1
  Sum2/1 -> Product/1
  Gain2/1 -> Sum3/1
  [v] -> Mux/1
  Demux/2 -> Unit Delay/1
  Discrete PID Controller/1 -> Gain2/1
  Discrete-Time Integrator3/1 -> Product2/1
  Product2/1 -> Sum4/1
  Constant1/1 -> Mux/3
  [wo] -> Sum3/2
  Mux/1 -> Alpha-Beta-Zero to dq1/1
  Sum1/1 -> Gain3/1, Gain/1
  Gain3/1 -> Discrete-Time Integrator3/1
  Alpha-Beta-Zero to dq1/1 -> Demux/1
  Constant2/1 -> [wo]
  Demux/3 -> Terminator1/1
  [qv] -> Mux/2
  Sum3/1 -> Integrator with Wrapped State (Discrete or Continuous)/1, [woi]
  Product/1 -> Discrete-Time Integrator/1
  vin/1 -> Sum1/2
  Sum4/1 -> Sum1/1
  Unit Delay/1 -> Discrete PID Controller/1

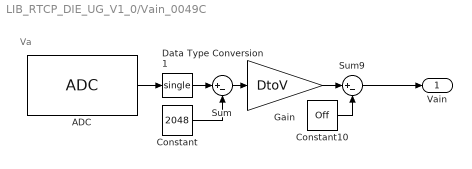
== system LIB_RTCP_DIE_UG_V1_0/Vain_0049C ==
  note: Va
  ADC : c2802xlib/ADC  blkParamProc=C2000_Type5  ADCModule=A  samplingMode=Single sample mode  ADCResolution=12-bit (Single-ended input)  useSOC1=SOC0  useSOC2=SOC0_SOC1  SOCAcquisitionWindow=AQPSv  SOCTriggerSource=Software  SOCInterruptTrigger=No ADCINT  Ts=Ts  dType=uint16  postInterrupt=off  interruptSel=ADCINT1  ADCINTContinuous=on  endma=off  chdma=1  conv1=ADCINA0  conv2=ADCINA0 and ADCINB0  conv1_Type4=ADCIN5  conv2_Type4=ADCIN0 and ADCIN1
  Constant : Constant  Value=2048
  Constant10 : Constant  Value=Off
  Data Type Conversion1 : DataTypeConversion  OutDataTypeStr=single
  Gain : Gain  Gain=DtoV
  Sum : Sum  Inputs=|+-
  Sum9 : Sum  Inputs=|+-
  Vain : Outport
  wires:
  Gain/1 -> Sum9/1
  Data Type Conversion1/1 -> Sum/1
  Constant/1 -> Sum/2
  Constant10/1 -> Sum9/2
  Sum/1 -> Gain/1
  Sum9/1 -> Vain/1
  ADC/1 -> Data Type Conversion1/1

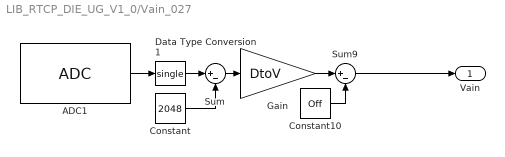
== system LIB_RTCP_DIE_UG_V1_0/Vain_027 ==
  ADC1 : c2802xlib/ADC  blkParamProc=C2000  ADCModule=1  samplingMode=Single sample mode  ADCResolution=12-bit (Single-ended input)  useSOC1=SOC0  useSOC2=SOC0_SOC1  SOCAcquisitionWindow=AQPSv  SOCTriggerSource=Software  SOCInterruptTrigger=No ADCINT  Ts=Ts  dType=uint16  postInterrupt=off  interruptSel=ADCINT1  ADCINTContinuous=on  endma=off  chdma=1  conv1=ADCINA7  conv2=ADCINA0 and ADCINB0  conv1_Type4=ADCIN0  conv2_Type4=ADCIN0 and ADCIN1
  Constant : Constant  Value=2048
  Constant10 : Constant  Value=Off
  Data Type Conversion1 : DataTypeConversion  OutDataTypeStr=single
  Gain : Gain  Gain=DtoV
  Sum : Sum  Inputs=|+-
  Sum9 : Sum  Inputs=|+-
  Vain : Outport
  wires:
  Gain/1 -> Sum9/1
  Data Type Conversion1/1 -> Sum/1
  Constant/1 -> Sum/2
  Constant10/1 -> Sum9/2
  Sum/1 -> Gain/1
  Sum9/1 -> Vain/1
  ADC1/1 -> Data Type Conversion1/1

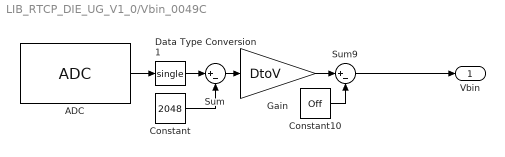
== system LIB_RTCP_DIE_UG_V1_0/Vbin_0049C ==
  ADC : c2802xlib/ADC  blkParamProc=C2000_Type5  ADCModule=B  samplingMode=Single sample mode  ADCResolution=12-bit (Single-ended input)  useSOC1=SOC0  useSOC2=SOC0_SOC1  SOCAcquisitionWindow=AQPSv  SOCTriggerSource=Software  SOCInterruptTrigger=No ADCINT  Ts=Ts  dType=uint16  postInterrupt=off  interruptSel=ADCINT1  ADCINTContinuous=on  endma=off  chdma=1  conv1=ADCINA0  conv2=ADCINA0 and ADCINB0  conv1_Type4=ADCIN0  conv2_Type4=ADCIN0 and ADCIN1
  Constant : Constant  Value=2048
  Constant10 : Constant  Value=Off
  Data Type Conversion1 : DataTypeConversion  OutDataTypeStr=single
  Gain : Gain  Gain=DtoV
  Sum : Sum  Inputs=|+-
  Sum9 : Sum  Inputs=|+-
  Vbin : Outport
  wires:
  Gain/1 -> Sum9/1
  Data Type Conversion1/1 -> Sum/1
  Constant/1 -> Sum/2
  Constant10/1 -> Sum9/2
  Sum/1 -> Gain/1
  Sum9/1 -> Vbin/1
  ADC/1 -> Data Type Conversion1/1

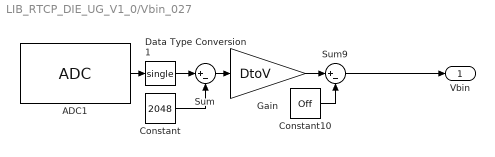
== system LIB_RTCP_DIE_UG_V1_0/Vbin_027 ==
  ADC1 : c2802xlib/ADC  blkParamProc=C2000  ADCModule=1  samplingMode=Single sample mode  ADCResolution=12-bit (Single-ended input)  useSOC1=SOC0  useSOC2=SOC0_SOC1  SOCAcquisitionWindow=AQPSv  SOCTriggerSource=Software  SOCInterruptTrigger=No ADCINT  Ts=Ts  dType=uint16  postInterrupt=off  interruptSel=ADCINT1  ADCINTContinuous=on  endma=off  chdma=1  conv1=ADCINA3  conv2=ADCINA0 and ADCINB0  conv1_Type4=ADCIN0  conv2_Type4=ADCIN0 and ADCIN1
  Constant : Constant  Value=2048
  Constant10 : Constant  Value=Off
  Data Type Conversion1 : DataTypeConversion  OutDataTypeStr=single
  Gain : Gain  Gain=DtoV
  Sum : Sum  Inputs=|+-
  Sum9 : Sum  Inputs=|+-
  Vbin : Outport
  wires:
  Gain/1 -> Sum9/1
  Data Type Conversion1/1 -> Sum/1
  Constant/1 -> Sum/2
  Constant10/1 -> Sum9/2
  Sum/1 -> Gain/1
  Sum9/1 -> Vbin/1
  ADC1/1 -> Data Type Conversion1/1

== system LIB_RTCP_DIE_UG_V1_0/Vcin_0049C ==
  ADC : c2802xlib/ADC  blkParamProc=C2000_Type5  ADCModule=C  samplingMode=Single sample mode  ADCResolution=12-bit (Single-ended input)  useSOC1=SOC0  useSOC2=SOC0_SOC1  SOCAcquisitionWindow=AQPSv  SOCTriggerSource=Software  SOCInterruptTrigger=No ADCINT  Ts=Ts  dType=uint16  postInterrupt=off  interruptSel=ADCINT1  ADCINTContinuous=on  endma=off  chdma=1  conv1=ADCINA0  conv2=ADCINA0 and ADCINB0  conv1_Type4=ADCIN2  conv2_Type4=ADCIN0 and ADCIN1
  Constant : Constant  Value=2048
  Constant10 : Constant  Value=Off
  Data Type Conversion1 : DataTypeConversion  OutDataTypeStr=single
  Gain : Gain  Gain=DtoV
  Sum : Sum  Inputs=|+-
  Sum9 : Sum  Inputs=|+-
  Vcin : Outport
  wires:
  Gain/1 -> Sum9/1
  Data Type Conversion1/1 -> Sum/1
  Constant/1 -> Sum/2
  Constant10/1 -> Sum9/2
  Sum/1 -> Gain/1
  Sum9/1 -> Vcin/1
  ADC/1 -> Data Type Conversion1/1

== system LIB_RTCP_DIE_UG_V1_0/Vcin_027 ==
  ADC1 : c2802xlib/ADC  blkParamProc=C2000  ADCModule=1  samplingMode=Single sample mode  ADCResolution=12-bit (Single-ended input)  useSOC1=SOC0  useSOC2=SOC0_SOC1  SOCAcquisitionWindow=AQPSv  SOCTriggerSource=Software  SOCInterruptTrigger=No ADCINT  Ts=Ts  dType=uint16  postInterrupt=off  interruptSel=ADCINT1  ADCINTContinuous=on  endma=off  chdma=1  conv1=ADCINA1  conv2=ADCINA0 and ADCINB0  conv1_Type4=ADCIN0  conv2_Type4=ADCIN0 and ADCIN1
  Constant : Constant  Value=2048
  Constant10 : Constant  Value=Off
  Data Type Conversion1 : DataTypeConversion  OutDataTypeStr=single
  Gain : Gain  Gain=DtoV
  Sum : Sum  Inputs=|+-
  Sum9 : Sum  Inputs=|+-
  Vcin : Outport
  wires:
  Gain/1 -> Sum9/1
  Data Type Conversion1/1 -> Sum/1
  Constant/1 -> Sum/2
  Constant10/1 -> Sum9/2
  Sum/1 -> Gain/1
  Sum9/1 -> Vcin/1
  ADC1/1 -> Data Type Conversion1/1
